simulink model "Simulazione_postura"  (R2020b)
settings: Solver=VariableStepAuto  StartTime=0.0  StopTime=10  RelTol=1e-3
InitFcn:
  | Inizializzazione
StopFcn:
  | visualizzazione
values from neighbouring files (symbols this model uses):
  R0 = [x0; y0; th0]    [Inizializzazione.m]
settings Model: Creator=andre  LastModifiedBy=andre

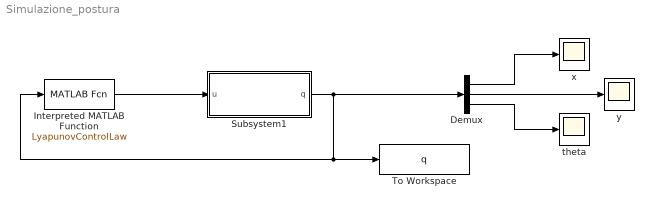
== system Simulazione_postura ==
  Demux : Demux  Outputs=3
  Interpreted MATLAB Function : MATLABFcn  MATLABFcn=LyapunovControlLaw
  Subsystem1 : Subsystem
  To Workspace : ToWorkspace  VariableName=q  SampleTime=-1
  theta : Scope
  x : Scope
  y : Scope
  wires:
  Interpreted MATLAB Function/1 -> Subsystem1/1(u)
  Demux/3 -> theta/1
  Demux/1 -> x/1
  Demux/2 -> y/1
  Subsystem1/1(q) -> To Workspace/1, Interpreted MATLAB Function/1, Demux/1

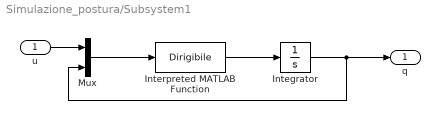
== system Simulazione_postura/Subsystem1 ==
  u : Inport
  Integrator : Integrator  InitialCondition=R0
  Interpreted MATLAB Function : MATLABFcn  MATLABFcn=Dirigibile
  Mux : Mux  Inputs=2
  q : Outport
  wires:
  Interpreted MATLAB Function/1 -> Integrator/1
  Mux/1 -> Interpreted MATLAB Function/1
  Integrator/1 -> q/1, Mux/2
  u/1 -> Mux/1
